simulink model "twosite_system_sampled"  (R2023a)
settings: Solver=ode45  StartTime=-180  StopTime=60*40  RelTol=1e-6
settings Model: Creator=hoshino  LastModifiedBy=hoshino
settings SolverCC: MaxConsecutiveMinStep=10  AlgebraicLoopSolver=TrustRegion
settings DebuggingCC: UnconnectedInputMsg=warning  UnconnectedOutputMsg=warning  UnconnectedLineMsg=warning
settings ModelReferenceCC: EnableRefExpFcnMdlSchedulingChecks=on
settings SFSimCC: CustomCodeUndefinedFunction=UseInterfaceOnly
settings RTWCC: DLArmComputeVersion=19.05

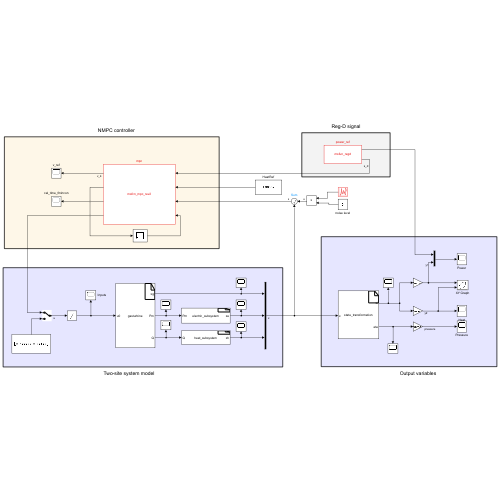
[thumbnail: Simulink's stored preview of the top-level diagram]
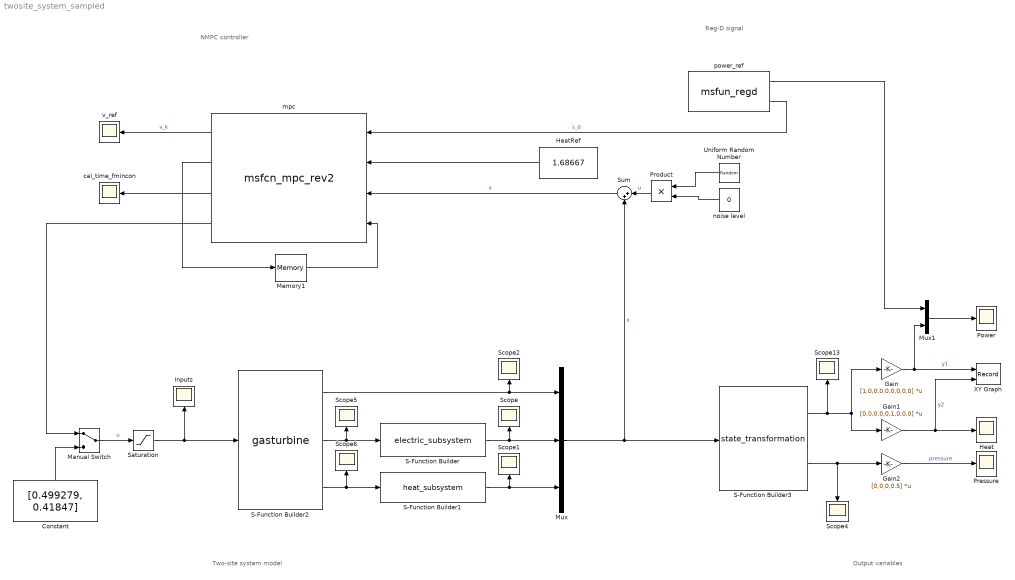
== system twosite_system_sampled ==
  note: Output variables
  note: Reg-D signal
  note: NMPC controller
  note: Two-site system model
  Constant : Constant  Value=[0.499279, 0.41847]
  Gain : Gain  Gain=[1,0,0,0,0,0,0,0,0]  Multiplication=Matrix(K*u) (u vector)
  Gain1 : Gain  Gain=[0,0,0,0,0,1,0,0,0]  Multiplication=Matrix(K*u) (u vector)
  Gain2 : Gain  Gain=[0,0,0,0.5]  Multiplication=Matrix(K*u) (u vector)
  Heat : Scope
  HeatRef : Constant  Value=1.68667
  Inputs : Scope
  Manual Switch : ManualSwitch
  Memory1 : Memory  InitialCondition=[1,1.69,1,1.69,1,1.69,1,1.69]  InheritSampleTime=on
  Mux : Mux  Inputs=3
  Mux1 : Mux  Inputs=2
  Power : Scope
  Pressure : Scope
  Product : Product
  S-Function Builder : S-Function  InitFcn=try, set_param(gcb,'FunctionName','electric_subsystem'), end  FunctionName=electric_subsystem  SFunctionModules=electric_subsystem_wrapper cforms  SFunctionDeploymentMode=off  EnableBusSupport=off  mask(S-Function Builder){}
      mask help: Simulink:masks:SFunctionBuilder_MD
      mask init:
      | val = [[.9  0.75 0.75 1 1 .9 .9 1]',[1 1 0.75 0.75 .9 .9 1 .9]'];try , sys = get_param(gcb,'SfunBuilderFcnName');if isempty(sys), sys = get_param(gcb,'FunctionName'); end,catch, sys = get_param(gcb,'FunctionName'); end
      settings: CopyFcn=set_param(gcbh,'LinkStatus','none')  PreSaveFcn=try, set_param(gcb,'FunctionName','electric_subsystem'), end  OpenFcn=sfunctionwizard(gcbh)
      mask Display: plot(val(:,1),val(:,2)),disp(sys), port_label('input',1,'Pm'), port_label('output',1,'xe')
  S-Function Builder1 : S-Function  InitFcn=try, set_param(gcb,'FunctionName','heat_subsystem'), end  FunctionName=heat_subsystem  SFunctionModules=heat_subsystem_wrapper cforms  SFunctionDeploymentMode=off  EnableBusSupport=off  mask(S-Function Builder){}
      mask help: Simulink:masks:SFunctionBuilder_MD
      mask init: same as twosite_system_sampled/S-Function Builder
      settings: CopyFcn=set_param(gcbh,'LinkStatus','none')  PreSaveFcn=try, set_param(gcb,'FunctionName','heat_subsystem'), end  OpenFcn=sfunctionwizard(gcbh)
      mask Display: plot(val(:,1),val(:,2)),disp(sys), port_label('input',1,'Q'), port_label('output',1,'xh')
  S-Function Builder2 : S-Function  InitFcn=try, set_param(gcb,'FunctionName','gasturbine'), end  FunctionName=gasturbine  SFunctionModules=gasturbine_wrapper cforms  SFunctionDeploymentMode=off  EnableBusSupport=off  mask(S-Function Builder){}
      mask help: Simulink:masks:SFunctionBuilder_MD
      mask init: same as twosite_system_sampled/S-Function Builder
      settings: CopyFcn=set_param(gcbh,'LinkStatus','none')  PreSaveFcn=try, set_param(gcb,'FunctionName','gasturbine'), end  OpenFcn=sfunctionwizard(gcbh)
      mask Display: plot(val(:,1),val(:,2)),disp(sys),port_label('input',1,'u0'),port_label('output',1,'xg'),port_label('output',2,'Pm'),port_label('output',3,'Q')
  S-Function Builder3 : S-Function  InitFcn=try, set_param(gcb,'FunctionName','state_transformation'), end  FunctionName=state_transformation  SFunctionModules=state_transformation_wrapper cforms  SFunctionDeploymentMode=off  EnableBusSupport=off  mask(S-Function Builder){}
      mask help: Simulink:masks:SFunctionBuilder_MD
      mask init: same as twosite_system_sampled/S-Function Builder
      settings: CopyFcn=set_param(gcbh,'LinkStatus','none')  PreSaveFcn=try, set_param(gcb,'FunctionName','state_transformation'), end  OpenFcn=sfunctionwizard(gcbh)
      mask Display: plot(val(:,1),val(:,2)),disp(sys),port_label('input',1,'x'),port_label('output',1,'xi'),port_label('output',2,'eta')
  Saturation : Saturate  UpperLimit=[1.0, 1.0]  LowerLimit=[0, 0]
  Scope{,1..2,4..6,13} (7 alike) : Scope
  Sum : Sum  Inputs=|++
  Uniform Random Number : UniformRandomNumber  SampleTime=2
  XY Graph : Record  FileSettingsInternal="{\"entries\":[{\"content\":{\"excelSettings\":{\"content\":{},\"type\":\"Streamout.ExcelSettings\"}},\"type\":\"Streamout.FileSettingStorage\",\"uuid\":\"\"}],\"packageUris\":[\"http:\\/\\/schema.mathworks.com\\/mf0\\/streamout_blocks\\/R2020a\"],\"version\":\"1.0\"}"  Layout=[1 1]  SignalsInternal="{\"entries\":[{\"content\":{\"signals\":[{\"content\":{\"blockPath\":[],\"dimensions\":[1],\"domain\":\"\",\"lineColor\":\"#a2142f\",\"plots\":[1],\"port\":1,\"signalID\":17,\"signalName\":\"y1\"},\"type\":\"RecordBlkView.Signal\",\"uuid\":\"\"},{\"content\":{\"blockPath\":[],\"dimensions\":[1],\"domain\":\"\",\"lineColor\":\"#139fff\",\"port\":2,\"signalID\":20,\"signalName\":\"y2\"},\"type\":\"RecordBlkView.Signal\",\"uuid\":\"\"}]},\"type\":\"RecordBlkView.InputSignals\",\"uuid\":\"\"}],\"packageUris\":[\"http:\\/\\/schema.mathworks.com\\/mf0\\/streamout_blocks\\/R2020a\"],\"version\":\"1.0\"}"  VisualizationBindings="{\"xyplotplugin\":{\"info\":[{\"series\":[],\"subplotID\":1}]}}"  CompatibilityTag=XY
  cal_time_fmincon : Scope
  mpc : M-S-Function  FunctionName=msfcn_mpc_rev2  Parameters=Tstep, Nhorizon, Qz, Rv, Plim, u1max, u2max  mask{Tstep=2.0, Nhorizon=5, Qz=blkdiag( 10, eye(4), 10, eye(3) ), Rv=0.01*eye(2), Plim=[-50, 50], u1max=1.0, u2max=1.0}
      mask prompts: Qz "WeightQ"; Rv "WeightR"
      mask DialogControl ParameterGroupVar Prompt: パラメーター
  noise level : Constant  Value=0
  power_ref : M-S-Function  FunctionName=msfun_regd  Parameters=Pnominal, ASamplitude  mask{Pnominal=1.0, ASamplitude=0.4}
      mask DialogControl ParameterGroupVar Prompt: パラメーター
  v_ref : Scope
  wires:
  S-Function Builder2/2 -> S-Function Builder/1, Scope5/1
  S-Function Builder2/3 -> S-Function Builder1/1, Scope6/1
  S-Function Builder2/1 -> Mux/1, Scope2/1
  S-Function Builder3/2 -> Gain2/1, Scope4/1
  S-Function Builder3/1 -> Gain/1, Gain1/1, Scope13/1
  power_ref/2 -> mpc/1  "s_d"
  Gain/1 -> XY Graph/1, Mux1/2  "y1"
  Gain1/1 -> Heat/1, XY Graph/2  "y2"
  Gain2/1 -> Pressure/1  "pressure"
  power_ref/1 -> Mux1/1
  Mux1/1 -> Power/1
  Sum/1 -> mpc/3  "x"
  Manual Switch/1 -> Saturation/1  "u"
  Constant/1 -> Manual Switch/2
  HeatRef/1 -> mpc/2
  Memory1/1 -> mpc/4
  mpc/1 -> v_ref/1  "v_k"
  mpc/2 -> Memory1/1
  mpc/3 -> cal_time_fmincon/1
  S-Function Builder/1 -> Mux/2, Scope/1
  mpc/4 -> Manual Switch/1
  Mux/1 -> S-Function Builder3/1, Sum/2  "x"
  Uniform Random Number/1 -> Product/1
  S-Function Builder1/1 -> Mux/3, Scope1/1
  noise level/1 -> Product/2
  Saturation/1 -> Inputs/1, S-Function Builder2/1
  Product/1 -> Sum/1  "u"
